simulink model "HIF_Grid_Model"  (R2025b)
settings: Solver=VariableStepAuto  StartTime=0.0  StopTime=0.2  RelTol=1e-3
libraries: fl_lib x7, nesl_utility x5, ee_lib x3
settings Model: Creator=Hasantha Rukshan  LastModifiedBy=Hasantha Rukshan
settings SFSimCC: SimTargetLang=C++  SimDLTargetLibrary=mkl-dnn

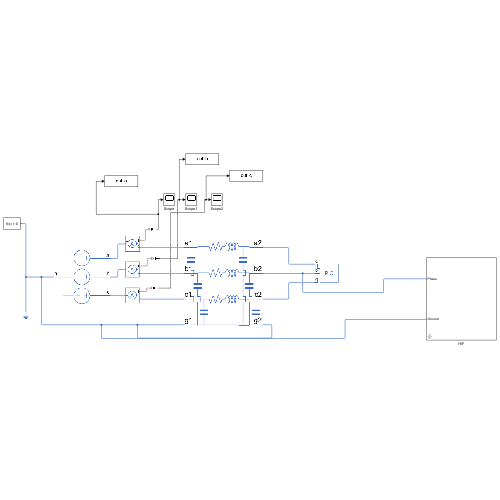
[thumbnail: Simulink's stored preview of the top-level diagram]
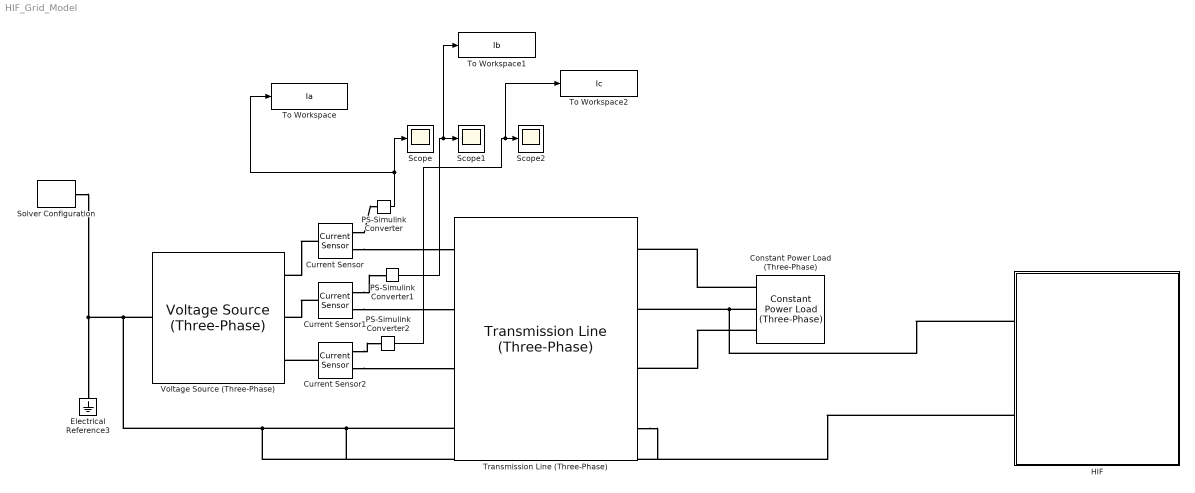
== system HIF_Grid_Model ==
  Constant Power Load (Three-Phase) : ee_lib/Passive/Constant Power Load (Three-Phase)  port_option=ee.enum.threePhasePort.expanded  FRated=50 Hz  active_power=500 kW  reactive_power=242 A*kV  Vline_rms_min=100 V  tau=0.01 s  Vline_rms_ini=11000 V  Vang_ini=0 deg  gmin=1e-6 S
      settings: InternalSimscapePortConfiguration="{\"Bottom\":[],\"Left\":[{\"id\":\"a\",\"label\":\"a\",\"type\":\"foundation.electrical.electrical\"},{\"id\":\"b\",\"label\":\"b\",\"type\":\"foundation.electrical.electrical\"},{\"id\":\"c\",\"label\":\"c\",\"type\":\"foundation.electrical.electrical\"}],\"Right\":[],\"Top\":[]}"
  Current Sensor : fl_lib/Electrical/Electrical Sensors/Current Sensor
  Current Sensor1 : fl_lib/Electrical/Electrical Sensors/Current Sensor
  Current Sensor2 : fl_lib/Electrical/Electrical Sensors/Current Sensor
  Electrical Reference3 : fl_lib/Electrical/Electrical Elements/Electrical Reference
  HIF : Subsystem  mask{FaultStartTime=0.1, FaultResistance=50, ArcNoiseAmplitude=50}
      mask prompts: FaultStartTime "Fault Start Time (s)"; FaultResistance "Fault Resistance (Ohms)"; ArcNoiseAmplitude "Arc Noise Amplitude"
  PS-Simulink Converter : nesl_utility/PS-Simulink Converter  PhysicalDomain=network_engine_domain  SubClassName=ps_output  LeftPortType=input  RightPortType=output  PseudoPeriodic=off  Frequencies=[]  VectorFormat=inherit  Unit=inherit  AffineConversion=off
  PS-Simulink Converter1 : nesl_utility/PS-Simulink Converter  PhysicalDomain=network_engine_domain  SubClassName=ps_output  LeftPortType=input  RightPortType=output  PseudoPeriodic=off  Frequencies=[]  VectorFormat=inherit  Unit=inherit  AffineConversion=off
  PS-Simulink Converter2 : nesl_utility/PS-Simulink Converter  PhysicalDomain=network_engine_domain  SubClassName=ps_output  LeftPortType=input  RightPortType=output  PseudoPeriodic=off  Frequencies=[]  VectorFormat=inherit  Unit=inherit  AffineConversion=off
  Scope : Scope
      settings: ActiveDisplayYMinimum=-805.52038735451015  ActiveDisplayYMaximum=550.00744546958
  Scope1 : Scope
      settings: ActiveDisplayYMinimum=-3.5532944456494704  ActiveDisplayYMaximum=408.28629745180132
  Scope2 : Scope
      settings: ActiveDisplayYMinimum=-108.62366943012151  ActiveDisplayYMaximum=142.44425369442467  DataLoggingVariableName=ScopeData2
  Solver Configuration : nesl_utility/Solver Configuration  PhysicalDomain=network_engine_domain  SubClassName=solver  LeftPortType=input  RightPortType=generic  Tones=[]  Harmonics=[]  SimulateNoise=off  Profile=off  UseLocalSampling=off  EnableSwitchedLinearOptims=on  FrequencyDomain=off  UseCCode=off  RelTol=0.001  AbsTol=0.001  MinStep=1e-09  ToWorkspace=off  RevertToSquareIcSolve=off  NumHomotopyIterations=100  PhasorMode=off  PhasorModeNumHarmonics=1  ConsistencySolver=NEWTON_XTOL_AFTER_FTOL  IndexReductionMethod=DerivativeReplacement  DoDC=off  ResidualTolerance=1e-09  ConsistencyTolSource=GLOBAL  ConsistencyAbsTol=0.001  ConsistencyRelTol=0.001  ConsistencyTolFactor=0.001  UseLocalSolver=off  LocalSolverChoice=NE_BACKWARD_EULER_ADVANCER  ResolveIndetEquations=on  FunctionEvalNumThread=1  LocalSolverSampleTime=0.001  DoFixedCost=off  MaxNonlinIter=3  MaxModeIter=2  ComputeImpulses=off  ImpulseIterations=2  LinearAlgebra=auto  LinearAlgebraNumThread=0  EquationFormulation=NE_TIME_EF  DelaysMemoryBudget=1024  AutomaticFiltering=on  FilteringTimeConstant=0.001  PartitionStorageMethod=AS_NEEDED  PartitionMemoryBudget=1024  PartitionMethod=ROBUST  MultibodyUseLocalSolver=off  MultibodyLocalSolverChoice=ODE1  MultibodyLocalSolverSampleTime=0.001
  To Workspace : ToWorkspace  VariableName=Ia  SampleTime=-1
  To Workspace1 : ToWorkspace  VariableName=Ib  SaveFormat=Timeseries  SampleTime=-1
  To Workspace2 : ToWorkspace  VariableName=Ic  SaveFormat=Timeseries  SampleTime=-1
  Transmission Line (Three-Phase) : ee_lib/Passive/Lines/Transmission Line (Three-Phase)  length=2 km  freq=50 Hz  R=5 Ohm/km  L=5 mH/km  M=1 mH/km  Cl=0.3 uF/km  Cg=0.1 uF/km  Rm=0 Ohm/km  ModelTwoSections=ee.enum.enable.no  N=1  InterfacePosition=0.5 km  N1sec=1  N2sec=1  Access_ground=ee.enum.enable.no  R_parasitic=1e-6 Ohm  G_parasitic=1e-6 1/Ohm
      settings: InternalSimscapePortConfiguration="{\"Bottom\":[],\"Left\":[{\"id\":\"a1\",\"label\":\"a1\",\"type\":\"foundation.electrical.electrical\"},{\"id\":\"b1\",\"label\":\"b1\",\"type\":\"foundation.electrical.electrical\"},{\"id\":\"c1\",\"label\":\"c1\",\"type\":\"foundation.electrical.electrical\"},{\"id\":\"g1\",\"label\":\"g1\",\"type\":\"foundation.electrical.electrical\"}],\"Right\":[{\"id\":\"a2\",\"label\":\"a2\",\"type\":\"foundation.electrical.electrical\"},{\"id\":\"b2\",\"label\":\"b2\",\"type\":\"foundation.electrical.electrical\"},{\"id\":\"c2\",\"label\":\"c2\",\"type\":\"foundation.electrical.electrical\"},{\"id\":\"g2\",\"label\":\"g2\",\"type\":\"foundation.electrical.electrical\"}],\"Top\":[]}"
  Voltage Source (Three-Phase) : ee_lib/Sources/Voltage Source (Three-Phase)  vline_rms=11000 V  shift=0 deg  freq=50 Hz  impedance_option=1  SShortCircuit=100e6 A*V  XR=15  R=0.01 Ohm  L=3.97e-4 H  harmonic_option=0  harmonic_orders=[5, 7, 11, 13]  harmonic_ratios=[.1, .1, .1, .1]  G_parasitic=0 1/Ohm  I_specify=off  I_priority=None  I=[0, 0, 0] A  I_nominal_specify=off  I_nominal_value=1  I_nominal_unit=A
      settings: InternalSimscapePortConfiguration="{\"Bottom\":[],\"Left\":[{\"id\":\"n\",\"label\":\"n\",\"type\":\"foundation.electrical.electrical\"}],\"Right\":[{\"id\":\"a\",\"label\":\"a\",\"type\":\"foundation.electrical.electrical\"},{\"id\":\"b\",\"label\":\"b\",\"type\":\"foundation.electrical.electrical\"},{\"id\":\"c\",\"label\":\"c\",\"type\":\"foundation.electrical.electrical\"}],\"Top\":[]}"
  wires:
  PS-Simulink Converter1/1 -> To Workspace1/1, Scope1/1
  PS-Simulink Converter2/1 -> To Workspace2/1, Scope2/1
  PS-Simulink Converter/1 -> To Workspace/1, Scope/1
  connections:
  Solver Configuration/RConn1 -- HIF/LConn2 -- Transmission Line (Three-Phase)/RConn4 -- Transmission Line (Three-Phase)/LConn4 -- Voltage Source (Three-Phase)/LConn1 -- Electrical Reference3/LConn1
  Current Sensor2/RConn2 -- Transmission Line (Three-Phase)/LConn3
  Current Sensor1/RConn2 -- Transmission Line (Three-Phase)/LConn2
  Current Sensor/RConn2 -- Transmission Line (Three-Phase)/LConn1
  Current Sensor/LConn1 -- Voltage Source (Three-Phase)/RConn1
  Current Sensor1/LConn1 -- Voltage Source (Three-Phase)/RConn2
  Current Sensor2/LConn1 -- Voltage Source (Three-Phase)/RConn3
  Current Sensor/RConn1 -- PS-Simulink Converter/LConn1
  Current Sensor1/RConn1 -- PS-Simulink Converter1/LConn1
  Current Sensor2/RConn1 -- PS-Simulink Converter2/LConn1
  Constant Power Load (Three-Phase)/LConn2 -- HIF/LConn1 -- Transmission Line (Three-Phase)/RConn2
  Constant Power Load (Three-Phase)/LConn1 -- Transmission Line (Three-Phase)/RConn1
  Constant Power Load (Three-Phase)/LConn3 -- Transmission Line (Three-Phase)/RConn3

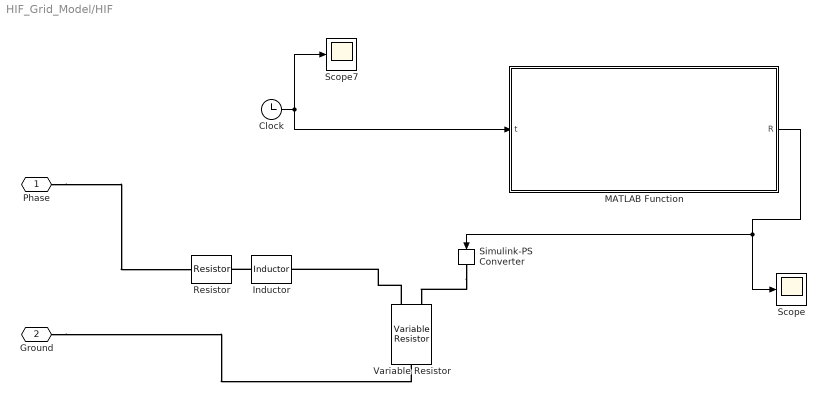
== system HIF_Grid_Model/HIF ==
  Clock : Clock
  Inductor : fl_lib/Electrical/Electrical Elements/Inductor  l=5e-3 H  r=0 Ohm  g=1e-9 1/Ohm  i_specify=off  i_priority=None  i=0 A  i_nominal_specify=off  i_nominal_value=1  i_nominal_unit=A  v_specify=off  v_priority=None  v=0 V  v_nominal_specify=off  v_nominal_value=1  v_nominal_unit=V  i_L_specify=off  i_L_priority=High  i_L=0 A  i_L_nominal_specify=off  i_L_nominal_value=1  i_L_nominal_unit=A
  MATLAB Function : MATLAB Function  TreatAsAtomicUnit=on
  Resistor : fl_lib/Electrical/Electrical Elements/Resistor  R=1 Ohm  i_specify=off  i_priority=None  i=0 A  i_nominal_specify=off  i_nominal_value=1  i_nominal_unit=A  v_specify=off  v_priority=None  v=0 V  v_nominal_specify=off  v_nominal_value=1  v_nominal_unit=V
  Scope : Scope
      settings: ActiveDisplayYMinimum=-7753.0395051754631  ActiveDisplayYMaximum=8090.8215276091923  DataLoggingVariableName=ScopeData3
  Scope7 : Scope
      settings: ActiveDisplayYMinimum=-0.025  ActiveDisplayYMaximum=0.225
  Simulink-PS Converter : nesl_utility/Simulink-PS Converter  PhysicalDomain=network_engine_domain  SubClassName=ps_input  LeftPortType=input  RightPortType=output  PseudoPeriodic=off  Frequencies=[]  NoiseDistribution=none  NoiseParameters=[]  Unit=Ohm  AffineConversion=off  FilteringAndDerivatives=provide  SimscapeFilterOrder=1  InputFilterTimeConstant=0.001  UdotUserProvided=0
  Variable Resistor : fl_lib/Electrical/Electrical Elements/Variable Resistor  Rmin=0 Ohm  thermalEnable=false  thermal_mass=1 J/K  i_specify=off  i_priority=None  i=0 A  i_nominal_specify=off  i_nominal_value=1  i_nominal_unit=A  v_specify=off  v_priority=None  v=0 V  v_nominal_specify=off  v_nominal_value=1  v_nominal_unit=V  T_specify=off  T_priority=None  T=300 K  T_nominal_specify=off  T_nominal_value=1  T_nominal_unit=K
  Phase : PMIOPort  Side=Left
  Ground : PMIOPort  Port=2  Side=Left
  wires:
  Clock/1 -> Scope7/1, MATLAB Function/1(t)
  MATLAB Function/1(R) -> Simulink-PS Converter/1, Scope/1
  connections:
  Variable Resistor/LConn2 -- Inductor/RConn1
  Inductor/LConn1 -- Resistor/RConn1
  Simulink-PS Converter/RConn1 -- Variable Resistor/LConn1
  Phase/RConn1 -- Resistor/LConn1
  Ground/RConn1 -- Variable Resistor/RConn1

== matlab function HIF_Grid_Model/HIF/MATLAB Function ==
  settings: updateMethod=DISCRETE
  data: t input; R output
function R = fault_resistance(t)

FaultStartTime = 0.1;

if t < FaultStartTime
    R = 1e6;
else
    if abs(sin(2*pi*50*t)) < 0.25
        R = 8000;   % arc OFF near zero crossing
    else
        R = 30;     % very low resistance when arc ON
    end
end
